simulink model "PointCloudTemplate"  (R2018b)
settings: Solver=VariableStepAuto  StartTime=0.0  StopTime=inf  RelTol=1e-3
PreLoadFcn:
  | % ROS setup
  | rosshutdown;
  | ipAddr = '';
  | rosinit(ipAddr)
  | 
  | % Sample times
  | sampleTime = 0.2;
  | 
  | % Control parameters
  | ctrlParam1 = 2;
  | ctrlParam2 = 3.5;
model workspace (MAT data in the model file):
  SL_ROS_VariableLengthArrays_MaxSizes.CommonInfo.ArrayTruncateAction = 'EmitWarning'
  SL_ROS_VariableLengthArrays_MaxSizes.MsgTypeMap = containers.Map
  SL_ROS_VariableLengthArrays_MaxSizes.MsgTypeMap.serialization.keys = {'sensor_msgs/PointCloud2'}
  SL_ROS_VariableLengthArrays_MaxSizes.MsgTypeMap.serialization.values{1}(1).PropertyName = 'Data'
  SL_ROS_VariableLengthArrays_MaxSizes.MsgTypeMap.serialization.values{1}(1).DataType = 'uint8'
  SL_ROS_VariableLengthArrays_MaxSizes.MsgTypeMap.serialization.values{1}(1).MaxLength = 9830400
  SL_ROS_VariableLengthArrays_MaxSizes.MsgTypeMap.serialization.values{1}(2).PropertyName = 'Fields'
  SL_ROS_VariableLengthArrays_MaxSizes.MsgTypeMap.serialization.values{1}(2).DataType = 'sensor_msgs/PointField'
  SL_ROS_VariableLengthArrays_MaxSizes.MsgTypeMap.serialization.values{1}(2).MaxLength = 16
  SL_ROS_VariableLengthArrays_MaxSizes.MsgTypeMap.serialization.uniformity = 0
  SL_ROS_VariableLengthArrays_MaxSizes.MsgTypeMap.serialization.keyType = 'char'
  SL_ROS_VariableLengthArrays_MaxSizes.MsgTypeMap.serialization.valueType = 'any'
undefined symbols (not defined in the file): gray, X, Y
libraries: robotlib x4, ROSPtCloudBlock x3
settings Model: Creator=scastro  LastModifiedBy=carlos
settings SFSimCC: SimUseLocalCustomCode=off
settings RTWCC: RTWUseLocalCustomCode=off

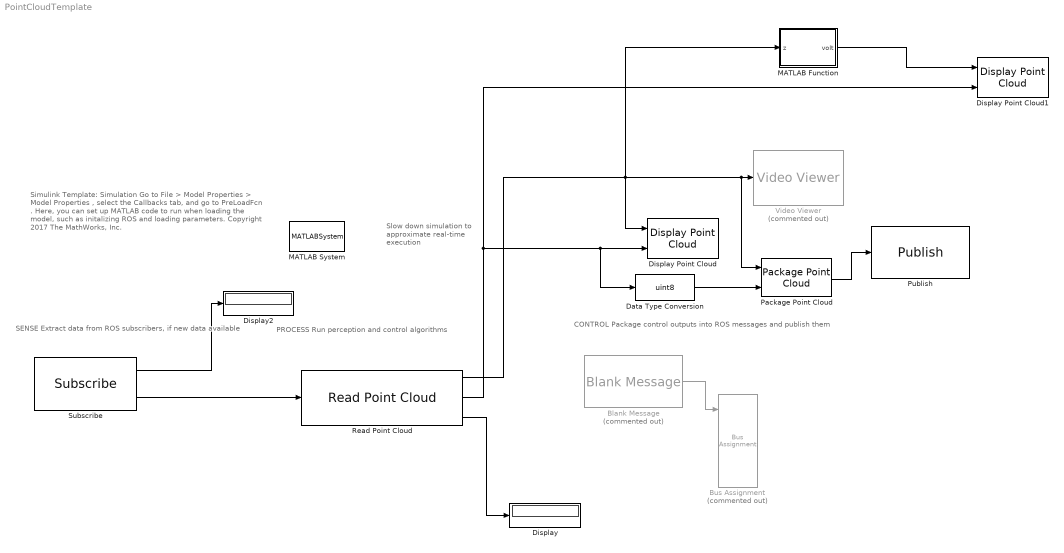
== system PointCloudTemplate ==
  note: Simulink Template: Simulation
      |
      | Go to File > Model Properties > Model Properties , select the Callbacks tab, and go to PreLoadFcn .
      |
      | Here, you can set up MATLAB code to run when loading the model, such as initalizing ROS and loading parameters.
      |
      | Copyright 2017 The MathWorks, Inc.
  note: Slow down simulation to approximate real-time execution
  note: PROCESS
      | Run perception and control algorithms
  note: SENSE
      | Extract data from ROS subscribers, if new data available
  note: CONTROL
      | Package control outputs into ROS messages and publish them
  Blank Message : robotlib/Blank Message  Commented=on  messageClass=Message  entityType=geometry_msgs/Point  messageType=geometry_msgs/Point  SampleTime=inf
      settings: SourceProductBaseCode=RO
  Bus Assignment : BusAssignment  Commented=on  AssignedSignals=X,Y
  Data Type Conversion : DataTypeConversion  OutDataTypeStr=uint8
  Display : Display
  Display Point Cloud : ROSPtCloudBlock/Display Point Cloud  xLimits=[-5 5]  yLimits=[-5 5]  zLimits=[-5 5]  maxSize=[480 640]
  Display Point Cloud1 : ROSPtCloudBlock/Display Point Cloud  xLimits=[-5 5]  yLimits=[-5 5]  zLimits=[-5 5]  maxSize=[480 640]
  Display2 : Display
  MATLAB Function : MATLAB Function  TreatAsAtomicUnit=on
  MATLAB System : MATLABSystem  System=ExampleHelperSimulationRateControl  SampleTime=sampleTime
      mask Type: ExampleHelperSimulationRateControl
      mask Display: disp('Rate Control');
  Package Point Cloud : ROSPtCloudBlock/Package Point Cloud  maxSize=[480 640]
  Publish : robotlib/Publish  topicSource=Specify your own  topic=/my_pub_topic  messageType=sensor_msgs/PointCloud2  messageQueueLength=1
      settings: SourceProductBaseCode=RO
  Read Point Cloud : robotlib/Read Point Cloud  MaximumPointCloudSize=[480, 640]  PreserveStructure=off  ShowRGBOutput=on  ShowIntensityOutput=off  ShowErrorCodeOutput=on  VariableSizeOutputs=off
      settings: SourceProductName=Robotics System Toolbox  SourceProductBaseCode=RO
  Subscribe : robotlib/Subscribe  topicSource=Select from ROS network  topic=/camera/depth_registered/points  messageType=sensor_msgs/PointCloud2  sampleTime=-1  messageQueueLength=1
      settings: SourceProductBaseCode=RO
  Video Viewer : VideoViewer  Commented=on  colormapValue=gray(256)  FigPos=[68 1078 1853 942]
  wires:
  Subscribe/2 -> Read Point Cloud/1
  Subscribe/1 -> Display2/1
  Blank Message/1 -> Bus Assignment/1
  Read Point Cloud/1 -> Package Point Cloud/1, Video Viewer/1, Display Point Cloud/1, MATLAB Function/1(z)
  Read Point Cloud/3 -> Display/1
  Read Point Cloud/2 -> Data Type Conversion/1, Display Point Cloud/2, Display Point Cloud1/2
  Package Point Cloud/1 -> Publish/1
  Data Type Conversion/1 -> Package Point Cloud/2
  MATLAB Function/1(volt) -> Display Point Cloud1/1

== matlab function PointCloudTemplate/MATLAB Function ==
  data: z input; volt output
function volt = SimpleKalman(z)

persistent A H Q R
persistent x P
persistent firstRun

if isempty(firstRun)
    A = 1;
    H=1;
    
    Q=0;
    R=4;
    
    x=14;
    P=6;
    
    firstRun=1;
end

xp=A*x;
Pp=A*P*A'+Q;

K=Pp*H'*inv(H*Pp*H'+R);

x=xp+K*(z-H*xp);
P=Pp-K*H*Pp;

volt=x;
